simulink model "TD_2order"  (R2019a)
settings: Solver=VariableStepAuto  StartTime=0.0  StopTime=10.0  RelTol=1e-3
libraries: dspsrcs4 x1
settings Model: Creator=jswl  LastModifiedBy=jswl

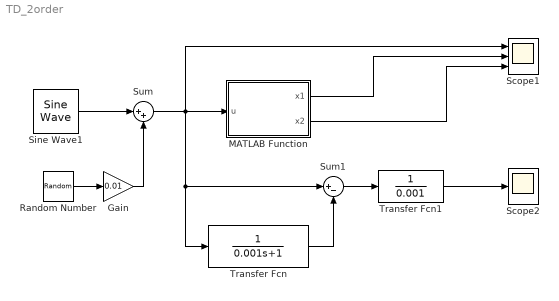
== system TD_2order ==
  Gain : Gain  Gain=0.01
  MATLAB Function : MATLAB Function  TreatAsAtomicUnit=on
  Random Number : RandomNumber  SampleTime=0.001
  Scope1 : Scope  NumInputPorts=3
  Scope2 : Scope
  Sine Wave1 : dspsrcs4/Sine Wave  Amplitude=1  Frequency=0.16  Phase=0  SampleMode=Discrete  OutComplex=Real  CompMethod=Trigonometric fcn  TableSize=Speed  SampleTime=0.001  SamplesPerFrame=1  ResetState=Restart at time zero  OutputFrames=off  dataType=double  wordLen=16  udDataType=sfix(16)  fracBitsMode=Best precision  numFracBits=15  OutDataTypeStr=double  LastOutDataTypeStr=double
  Sum : Sum  Inputs=|++
  Sum1 : Sum  Inputs=|+-
  Transfer Fcn : TransferFcn  Denominator=[0.001 1]
  Transfer Fcn1 : TransferFcn  Denominator=[0 0.001]
  wires:
  Random Number/1 -> Gain/1
  Sine Wave1/1 -> Sum/1
  Gain/1 -> Sum/2
  Sum/1 -> Scope1/1, Transfer Fcn/1, Sum1/1, MATLAB Function/1(u)
  MATLAB Function/1(x1) -> Scope1/2
  Transfer Fcn/1 -> Sum1/2
  Sum1/1 -> Transfer Fcn1/1
  MATLAB Function/2(x2) -> Scope1/3
  Transfer Fcn1/1 -> Scope2/1

== matlab function TD_2order/MATLAB Function ==
  data: u input; x1 output; x2 output
function [x1,x2] = TD_2order(u)
T=0.001;
r=20;
h=0.001;
persistent x_1 x_2
if isempty(x_1)
    x_1=u;
    x_2=0;
end
x1k=x_1;
x2k=x_2;
x_1=x1k+T*x2k;
x_2=x2k+T*fst(x1k,x2k,u,r,h);
x1=x_1;
x2=x_2;
end

function f=fst(x1,x2,u,r,h)
d=r*h;			%h为滤波因子  r为调节系数，r越大跟踪效果越好，但微分信号会增加高频噪声
d0=d*h;	%反之，微分信号越平滑，会产生一定的滞后
y=x1-u+h*x2;
a0=sqrt(d^2+8*r*abs(y));
if abs(y)<=d0
    a=x2+y/h;
else
    a=x2+0.5*(a0-d)*sign(y);
end
if abs(a)<=d
    f=-r*a/d;
else
    f=-r*sign(a);
end
end
